simulink model "RTC_DS3231_Demo"  (R2024b)
settings: Solver=FixedStepAuto  StartTime=0.0  StopTime=10.0  FixedStep=1.0  RelTol=1e-3
settings Model: Creator=Shreyas  LastModifiedBy=Shreyas
settings SFSimCC: SimCustomSourceCode="#include \"ds3231.c\""  SimCustomHeaderCode="#include \"ds3231.h\""
settings RTWCC: CustomSourceCode="#include \"ds3231.c\""  CustomHeaderCode="#include \"ds3231.h\""

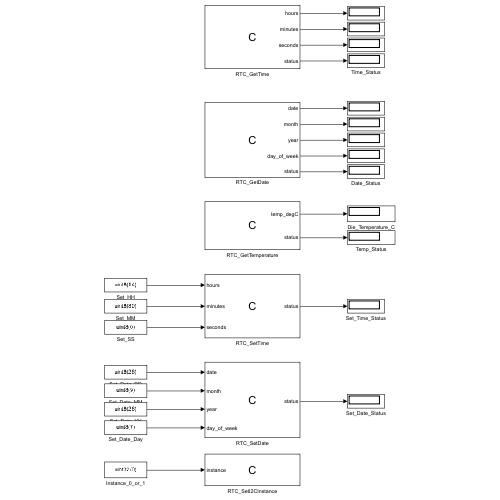
[thumbnail: Simulink's stored preview of the top-level diagram]
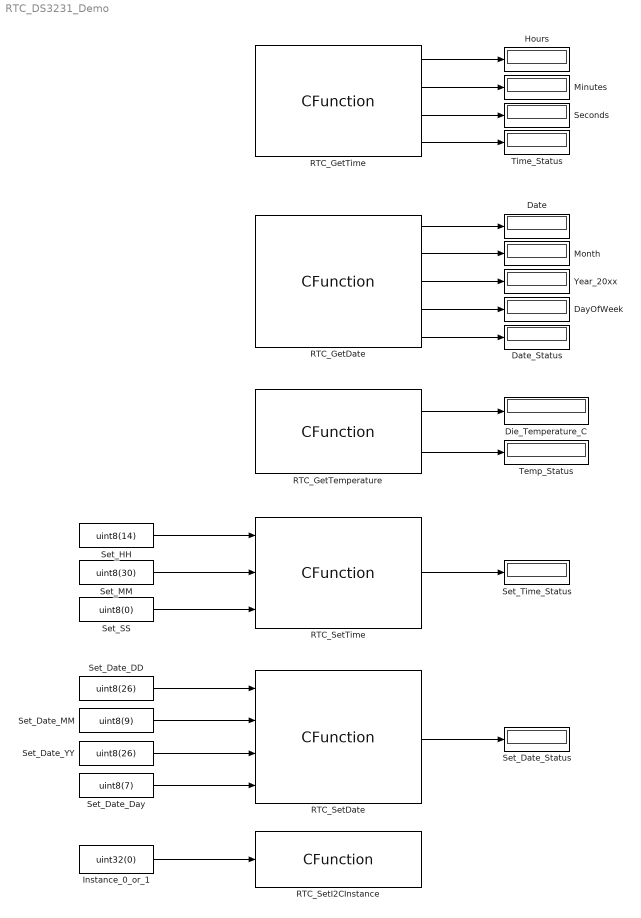
== system RTC_DS3231_Demo ==
  Date : Display
  Date_Status : Display
  DayOfWeek : Display
  Die_Temperature_C : Display
  Hours : Display
  Instance_0_or_1 : Constant  Value=uint32(0)  OutDataTypeStr=uint32
  Minutes : Display
  Month : Display
  RTC_GetDate : CFunction  OutputCode=|  CodegenOutputCode=|  SimCustomHeaderFile=ds3231.h  SimCustomSourceFile=ds3231.c  CustomHeaderFile=ds3231.h  CustomSourceFile=ds3231.c  CustomCodeIsMultiInstantiable=on
      OutputCode=|
      | /* Read Date: Date (1-31), Month (1-12), Year (0-99), DayOfWeek (1-7) */
      | status = DS3231_GetDateScalars(&year, &month, &date, &day_of_week);
      CodegenOutputCode=|
      | /* Read Date: Date (1-31), Month (1-12), Year (0-99), DayOfWeek (1-7) */
      | status = DS3231_GetDateScalars(&year, &month, &date, &day_of_week);
  RTC_GetTemperature : CFunction  OutputCode=|  CodegenOutputCode=|  SimCustomHeaderFile=ds3231.h  SimCustomSourceFile=ds3231.c  CustomHeaderFile=ds3231.h  CustomSourceFile=ds3231.c  CustomCodeIsMultiInstantiable=on
      OutputCode=|
      | /* Read Temperature: 0.25 degC resolution */
      | status = DS3231_GetTemperature(&temp_degC);
      CodegenOutputCode=|
      | /* Read Temperature: 0.25 degC resolution */
      | status = DS3231_GetTemperature(&temp_degC);
  RTC_GetTime : CFunction  OutputCode=|  CodegenOutputCode=|  SimCustomHeaderFile=ds3231.h  SimCustomSourceFile=ds3231.c  CustomHeaderFile=ds3231.h  CustomSourceFile=ds3231.c  CustomCodeIsMultiInstantiable=on
      OutputCode=|
      | /* Read Time: Hours (0-23), Minutes (0-59), Seconds (0-59) */
      | status = DS3231_GetTimeScalars(&hours, &minutes, &seconds);
      CodegenOutputCode=|
      | /* Read Time: Hours (0-23), Minutes (0-59), Seconds (0-59) */
      | status = DS3231_GetTimeScalars(&hours, &minutes, &seconds);
  RTC_SetDate : CFunction  OutputCode=|  CodegenOutputCode=|  SimCustomHeaderFile=ds3231.h  SimCustomSourceFile=ds3231.c  CustomHeaderFile=ds3231.h  CustomSourceFile=ds3231.c  CustomCodeIsMultiInstantiable=on
      OutputCode=|
      | /* Write Date to DS3231 */
      | status = DS3231_SetDateScalars(year, month, date, day_of_week);
      CodegenOutputCode=|
      | /* Write Date to DS3231 */
      | status = DS3231_SetDateScalars(year, month, date, day_of_week);
  RTC_SetI2CInstance : CFunction  OutputCode=|  CodegenOutputCode=|  SimCustomHeaderFile=ds3231.h  SimCustomSourceFile=ds3231.c  CustomHeaderFile=ds3231.h  CustomSourceFile=ds3231.c  CustomCodeIsMultiInstantiable=on
      OutputCode=|
      | /* Set LPI2C Hardware Instance (0 = LPI2C0, 1 = LPI2C1) */
      | DS3231_SetI2CInstance(instance);
      CodegenOutputCode=|
      | /* Set LPI2C Hardware Instance (0 = LPI2C0, 1 = LPI2C1) */
      | DS3231_SetI2CInstance(instance);
  RTC_SetTime : CFunction  OutputCode=|  CodegenOutputCode=|  SimCustomHeaderFile=ds3231.h  SimCustomSourceFile=ds3231.c  CustomHeaderFile=ds3231.h  CustomSourceFile=ds3231.c  CustomCodeIsMultiInstantiable=on
      OutputCode=|
      | /* Write Time to DS3231 */
      | status = DS3231_SetTimeScalars(hours, minutes, seconds);
      CodegenOutputCode=|
      | /* Write Time to DS3231 */
      | status = DS3231_SetTimeScalars(hours, minutes, seconds);
  Seconds : Display
  Set_Date_DD : Constant  Value=uint8(26)  OutDataTypeStr=uint8
  Set_Date_Day : Constant  Value=uint8(7)  OutDataTypeStr=uint8
  Set_Date_MM : Constant  Value=uint8(9)  OutDataTypeStr=uint8
  Set_Date_Status : Display
  Set_Date_YY : Constant  Value=uint8(26)  OutDataTypeStr=uint8
  Set_HH : Constant  Value=uint8(14)  OutDataTypeStr=uint8
  Set_MM : Constant  Value=uint8(30)  OutDataTypeStr=uint8
  Set_SS : Constant  Value=uint8(0)  OutDataTypeStr=uint8
  Set_Time_Status : Display
  Temp_Status : Display
  Time_Status : Display
  Year_20xx : Display
  wires:
  RTC_GetTime/1 -> Hours/1
  RTC_GetTime/2 -> Minutes/1
  RTC_GetTime/3 -> Seconds/1
  RTC_GetTime/4 -> Time_Status/1
  RTC_GetDate/1 -> Date/1
  RTC_GetDate/2 -> Month/1
  RTC_GetDate/3 -> Year_20xx/1
  RTC_GetDate/4 -> DayOfWeek/1
  RTC_GetDate/5 -> Date_Status/1
  RTC_GetTemperature/1 -> Die_Temperature_C/1
  RTC_GetTemperature/2 -> Temp_Status/1
  Set_HH/1 -> RTC_SetTime/1
  Set_MM/1 -> RTC_SetTime/2
  Set_SS/1 -> RTC_SetTime/3
  RTC_SetTime/1 -> Set_Time_Status/1
  Set_Date_DD/1 -> RTC_SetDate/1
  Set_Date_MM/1 -> RTC_SetDate/2
  Set_Date_YY/1 -> RTC_SetDate/3
  Set_Date_Day/1 -> RTC_SetDate/4
  RTC_SetDate/1 -> Set_Date_Status/1
  Instance_0_or_1/1 -> RTC_SetI2CInstance/1
